simulink model "Logical"  (Simulink 5.0)
settings: Solver=FixedStepDiscrete  StartTime=0.0  StopTime=10.0  RelTol=1e-3
settings Model: Creator=sofronis  LastModifiedBy=sofronis  ExtModeAutoUpdateStatusClock=off  AlgebraicLoopMsg=error

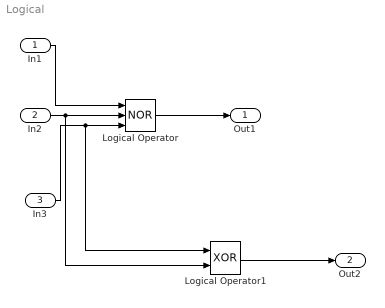
== system Logical ==
  In1 : Inport  SampleTime=1
  In2 : Inport  Port=2  SampleTime=1
  In3 : Inport  Port=3  SampleTime=1
  Logical Operator : Logic  Operator=NOR  Inputs=3  ShowAdditionalParam=on
  Logical Operator1 : Logic  Operator=XOR  ShowAdditionalParam=on
  Out1 : Outport
  Out2 : Outport  Port=2
  wires:
  In1/1 -> Logical Operator/1
  In2/1 -> Logical Operator/2, Logical Operator1/2
  Logical Operator/1 -> Out1/1
  In3/1 -> Logical Operator/3, Logical Operator1/1
  Logical Operator1/1 -> Out2/1
